simulink model "sigmoidFunc"  (R2021a)
settings: Solver=VariableStepAuto  StartTime=0.0  StopTime=10.0  RelTol=1e-3
libraries: simulink x1
settings Model: Creator=z_zha  LastModifiedBy=z_zha

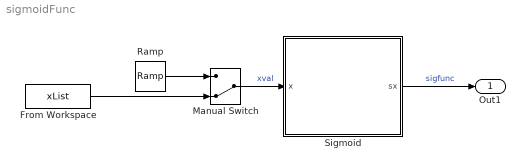
== system sigmoidFunc ==
  From Workspace : FromWorkspace  VariableName=xList
  Manual Switch : ManualSwitch  CurrentSetting=0
  Ramp : simulink/Sources/Ramp  slope=2  start=-5  InitialOutput=0
  Sigmoid : Subsystem  mask(Sigmoid){b=0.5, a=2}
      mask prompts: b "Input scale factor'b'"; a "Function range factor'a'"
      mask help:
      | An improved sigmoid function module, where the parameter 'a' and 'b' determine the function scale and input stretch. The formula as follows:
      |
      | s(x) = a[(1+e^{-bx})^{-1} - .5]
  Out1 : Outport
  wires:
  Manual Switch/1 -> Sigmoid/1(x)  "xval"
  From Workspace/1 -> Manual Switch/2
  Ramp/1 -> Manual Switch/1
  Sigmoid/1(sx) -> Out1/1  "sigfunc"

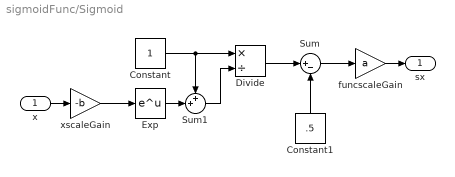
== system sigmoidFunc/Sigmoid ==
  x : Inport
  Constant : Constant
  Constant1 : Constant  Value=.5
  Divide : Product  Inputs=*/
  Exp : Math  SaturateOnIntegerOverflow=on
  Sum : Sum  Inputs=|+-
  Sum1 : Sum  Inputs=++|
  funcscaleGain : Gain  Gain=a
  xscaleGain : Gain  Gain=-b
  sx : Outport
  wires:
  Divide/1 -> Sum/1
  x/1 -> xscaleGain/1
  Constant/1 -> Sum1/1, Divide/1
  xscaleGain/1 -> Exp/1
  Constant1/1 -> Sum/2
  Sum/1 -> funcscaleGain/1
  funcscaleGain/1 -> sx/1
  Exp/1 -> Sum1/2
  Sum1/1 -> Divide/2
